simulink model "temp_heat1"  (R2024b)
settings: Solver=VariableStepAuto  StartTime=0.0  StopTime=1000  RelTol=1e-3
settings Model: Creator=shiva  LastModifiedBy=shiva

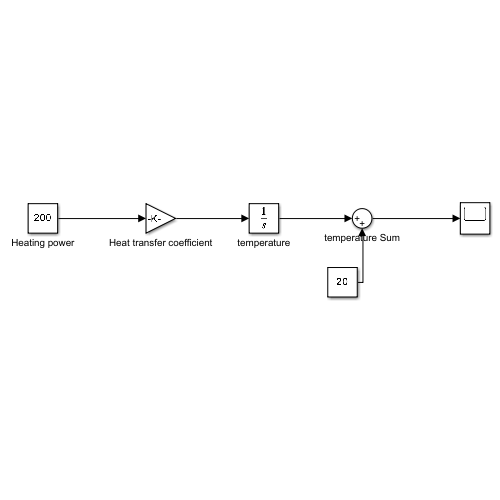
[thumbnail: Simulink's stored preview of the top-level diagram]
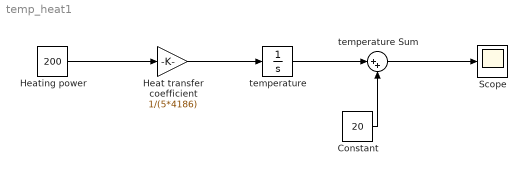
== system temp_heat1 ==
  Constant : Constant  Value=20
  Heat transfer coefficient : Gain  Gain=1/(5*4186)
  Heating power : Constant  Value=200
  Scope : Scope
  temperature : Integrator  InitialCondition=20
  temperature Sum : Sum  Inputs=|++
  wires:
  Heating power/1 -> Heat transfer coefficient/1
  Heat transfer coefficient/1 -> temperature/1
  Constant/1 -> temperature Sum/2
  temperature/1 -> temperature Sum/1
  temperature Sum/1 -> Scope/1
